simulink model "Feedforward_demo_Feb25_2017"  (R2016a)
settings: Solver=ode4  StartTime=0.0  StopTime=5  FixedStep=0.0001  RelTol=1e-3
values from neighbouring files (symbols this model uses):
  k = 10    [ff_demo_set_up.m]
  Kf = 1/(p+k)    (= 0.0666666666667)    [ff_demo_set_up.m]
  p = 5    [ff_demo_set_up.m]
libraries: simulink x4
settings Model: Creator=tac29  LastModifiedBy=DR_C

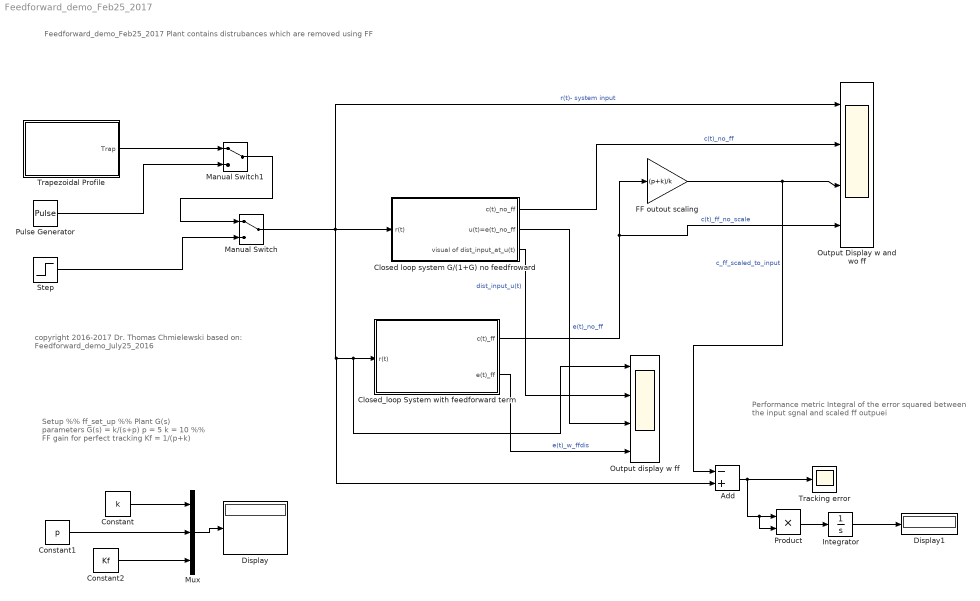
== system Feedforward_demo_Feb25_2017 ==
  note: Feedforward_demo_Feb25_2017
      | Plant contains distrubances which are removed using FF
  note: Performance metric
      | Integral of the error squared between
      | the input sgnal and scaled ff outpuei
  note: Setup
      | %% ff_set_up
      | %% Plant G(s) parameters   G(s) = k/(s+p)
      | p = 5
      | k = 10
      |
      | %% FF gain for perfect tracking
      | Kf = 1/(p+k)
  note: copyright 2016-2017
      | Dr. Thomas Chmielewski
      | based on:
      | Feedforward_demo_July25_2016
  Add : Sum  Inputs=-+
  Closed loop system G/(1+G) no feedfroward : Subsystem
  Closed_loop System with feedforward term : Subsystem
  Constant : Constant  Value=k
  Constant1 : Constant  Value=p
  Constant2 : Constant  Value=Kf
  Display : Display
  Display1 : Display
  FF outout scaling : Gain  Gain=(p+k)/k
  Integrator : Integrator
  Manual Switch : ManualSwitch
  Manual Switch1 : ManualSwitch
  Mux : Mux  Inputs=3
  Output Display w and wo ff : Scope  NumInputPorts=4
  Output display w ff : Scope  NumInputPorts=4
  Product : Product
  Pulse Generator : DiscretePulseGenerator  PulseType=Time based  Period=1  PulseWidth=50
  Step : Step  Time=0  SampleTime=0
  Tracking error : Scope
  Trapezoidal Profile : Subsystem
  wires:
  Step/1 -> Manual Switch/2
  Manual Switch/1 -> Output Display w and wo ff/1, Add/2, Output display w ff/1, Closed_loop System with feedforward term/1(r(t)), Closed loop system G/(1+G) no feedfroward/1(r(t))  "r(t)- system input"
  Mux/1 -> Display/1
  Constant2/1 -> Mux/3
  Constant1/1 -> Mux/2
  Constant/1 -> Mux/1
  FF outout scaling/1 -> Add/1, Output Display w and wo ff/3  "c_ff_scaled_to_input"
  Manual Switch1/1 -> Manual Switch/1
  Pulse Generator/1 -> Manual Switch1/2
  Closed loop system G/(1+G) no feedfroward/1(c(t)_no_ff) -> Output Display w and wo ff/2  "c(t)_no_ff"
  Closed_loop System with feedforward term/1(c(t)_ff) -> FF outout scaling/1, Output Display w and wo ff/4  "c(t)_ff_no_scale"
  Add/1 -> Product/2, Product/1, Tracking error/1
  Product/1 -> Integrator/1
  Integrator/1 -> Display1/1
  Closed loop system G/(1+G) no feedfroward/2(u(t)=e(t)_no_ff) -> Output display w ff/3  "e(t)_no_ff"
  Closed_loop System with feedforward term/2(e(t)_ff) -> Output display w ff/4  "e(t)_w_ffdis"
  Closed loop system G/(1+G) no feedfroward/3(visual of dist_input_at_u(t)) -> Output display w ff/2  "dist_input_u(t)"
  Trapezoidal Profile/1(Trap) -> Manual Switch1/1

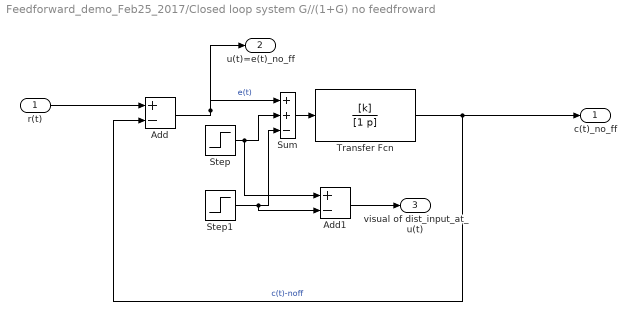
== system Feedforward_demo_Feb25_2017/Closed loop system G//(1+G) no feedfroward ==
  r(t) : Inport
  Add : Sum  Inputs=+-
  Add1 : Sum  Inputs=+-
  Step : Step  Time=1.5  SampleTime=0
  Step1 : Step  Time=1.6  SampleTime=0
  Sum : Sum  Inputs=|++-
  Transfer Fcn : TransferFcn  Numerator=[k]  Denominator=[1 p]
  c(t)_no_ff : Outport
  u(t)=e(t)_no_ff : Outport  Port=2
  visual of dist_input_at_u(t) : Outport  Port=3
  wires:
  Transfer Fcn/1 -> Add/2, c(t)_no_ff/1  "c(t)-noff"
  Add/1 -> u(t)=e(t)_no_ff/1, Sum/1  "e(t)"
  r(t)/1 -> Add/1
  Sum/1 -> Transfer Fcn/1
  Step/1 -> Add1/1, Sum/2
  Step1/1 -> Add1/2, Sum/3
  Add1/1 -> visual of dist_input_at_u(t)/1

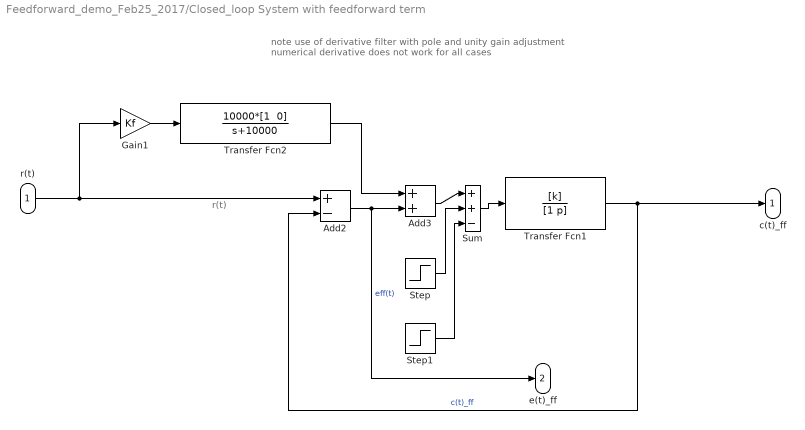
== system Feedforward_demo_Feb25_2017/Closed_loop System with feedforward term ==
  note: note use of derivative filter with pole and unity gain adjustment
      | numerical derivative does not work for all cases
  note: r(t)
  r(t) : Inport
  Add2 : Sum  Inputs=+-
  Add3 : Sum
  Gain1 : Gain  Gain=Kf
  Step : Step  Time=0  SampleTime=0
  Step1 : Step  Time=0  SampleTime=0
  Sum : Sum  Inputs=|++-
  Transfer Fcn1 : TransferFcn  Numerator=[k]  Denominator=[1 p]
  Transfer Fcn2 : TransferFcn  Numerator="10000*[1  0]"  Denominator=[1 10000]
  c(t)_ff : Outport
  e(t)_ff : Outport  Port=2
  wires:
  Add2/1 -> e(t)_ff/1, Add3/2  "eff(t)"
  Gain1/1 -> Transfer Fcn2/1
  Transfer Fcn1/1 -> c(t)_ff/1, Add2/2  "c(t)_ff"
  Transfer Fcn2/1 -> Add3/1
  r(t)/1 -> Add2/1, Gain1/1
  Add3/1 -> Sum/1
  Sum/1 -> Transfer Fcn1/1
  Step/1 -> Sum/2
  Step1/1 -> Sum/3

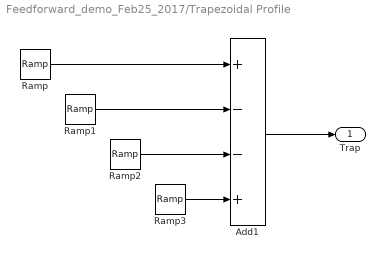
== system Feedforward_demo_Feb25_2017/Trapezoidal Profile ==
  Add1 : Sum  Inputs=+--+
  Ramp : simulink/Sources/Ramp  slope=1  start=0  X0=0
  Ramp1 : simulink/Sources/Ramp  slope=1  start=1  X0=0
  Ramp2 : simulink/Sources/Ramp  slope=1  start=2  X0=0
  Ramp3 : simulink/Sources/Ramp  slope=1  start=3  X0=0
  Trap : Outport
  wires:
  Ramp/1 -> Add1/1
  Ramp3/1 -> Add1/4
  Ramp2/1 -> Add1/3
  Ramp1/1 -> Add1/2
  Add1/1 -> Trap/1
